simulink model "UndampedOscillator_Estimator"  (R2020a)
settings: Solver=ode4  StartTime=0.0  StopTime=6  FixedStep=0.001  RelTol=1e-3
settings Model: Creator=XShen  LastModifiedBy=Shen
settings DataIOCC: ReturnWorkspaceOutputs=off
settings DebuggingCC: ArithmeticOperatorsInVariantConditions=warning
settings SFSimCC: SimUseLocalCustomCode=off  CustomCodeUndefinedFunction=UseInterfaceOnly
settings RTWCC: RTWUseLocalCustomCode=off
settings CodeAppCC: StateflowObjectComments=on

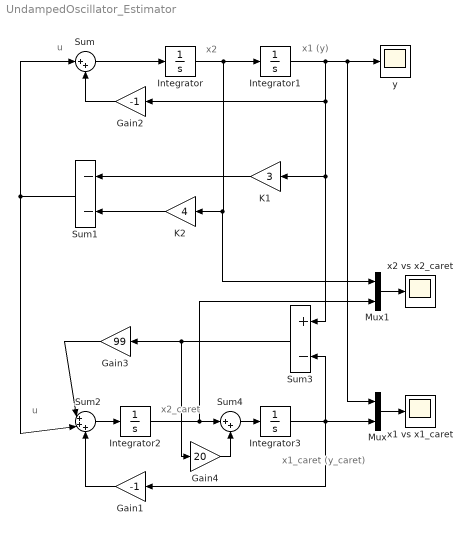
== system UndampedOscillator_Estimator ==
  note: u
  note: x1 (y)
  note: x2
  note: x1_caret
      | (y_caret)
  note: x2_caret
  note: u
  Gain1 : Gain  Gain=-1
  Gain2 : Gain  Gain=-1
  Gain3 : Gain  Gain=99
  Gain4 : Gain  Gain=20
  Integrator : Integrator
  Integrator1 : Integrator  InitialCondition=2
  Integrator2 : Integrator  InitialCondition=-2
  Integrator3 : Integrator
  K1 : Gain  Gain=3
  K2 : Gain  Gain=4
  Mux : Mux  Inputs=2
  Mux1 : Mux  Inputs=2
  Sum : Sum  Inputs=|++
  Sum1 : Sum  Inputs=--
  Sum2 : Sum  Inputs=|+++
  Sum3 : Sum  Inputs=+-
  Sum4 : Sum  Inputs=|++
  x1 vs x1_caret : Scope
  x2 vs x2_caret : Scope
  y : Scope
  wires:
  Integrator/1 -> Mux1/1, K2/1, Integrator1/1
  Integrator1/1 -> Mux/1, y/1, Gain2/1, Sum3/1, K1/1
  Sum/1 -> Integrator/1
  Gain2/1 -> Sum/2
  Sum1/1 -> Sum2/2, Sum/1
  Integrator3/1 -> Mux/2, Sum3/2, Gain1/1
  Sum2/1 -> Integrator2/1
  K1/1 -> Sum1/1
  K2/1 -> Sum1/2
  Sum3/1 -> Gain4/1, Gain3/1
  Gain1/1 -> Sum2/3
  Gain3/1 -> Sum2/1
  Sum4/1 -> Integrator3/1
  Gain4/1 -> Sum4/2
  Mux/1 -> x1 vs x1_caret/1
  Integrator2/1 -> Mux1/2, Sum4/1
  Mux1/1 -> x2 vs x2_caret/1
